simulink model "TRN_test"  (R2022a)
settings: Solver=FixedStepDiscrete  StartTime=0.0  StopTime=300  FixedStep=0.04  RelTol=1e-3
PreLoadFcn:
  | listing = dir;
  | if (contains([listing .name], 'FLCC')) && (contains([listing .name], 'DYN'))
  |     addpath('./DYN', './FLCC', './FTG', './GPS', './INS', './MAP', './RALT', '../TRN');
  | elseif (contains([listing .name], 'FTG.slx'))
  |     addpath('../DYN', '../FLCC', '../FTG', '../GPS', '../INS', '../MAP', '../RALT', '../TRN');
  | else
  | 
  | end
  | 
  | load('BUS_STRUCTURE_DYN.mat');
  | load('BUS_STRUCTURE_FLCC.mat');
  | load('BUS_STRUCTURE_RALT.mat');
  | load('BUS_STRUCTURE_INS.mat');
  | load('BUS_STRUCTURE_GPS.mat');
  | FTG_initState;
  | 
  | addpath('C:/MAP2');
InitFcn:
  | addpath('C:/MAP2');
  | load('BusStructureTRN.mat');
model workspace (MAT data in the model file):
  initLLA = [0 0 0]
libraries: aerolibconvert2 x14, simulink_extras x8
settings Model: ParameterArgumentNames=initLLA  Creator=HSU  LastModifiedBy=JSLee
settings SolverCC: AlgebraicLoopSolver=TrustRegion
settings DataIOCC: ExternalInput=FTGScenario.getElement('IN_STICK'),[],[],FTGScenario.getElement('IN_FLIGHT_CMD'),[]  LoadExternalInput=on  SaveOutput=off  DSMLogging=off  SaveTime=off
settings OptimizationCC: BlockReduction=off  DefaultParameterBehavior=Inlined  UseDivisionForNetSlopeComputation=on  GainParamInheritBuiltInType=on  UseFloatMulNetSlope=on  InlineInvariantSignals=on  EnhancedBackFolding=on  PassReuseOutputArgsAs=Individual arguments  ZeroExternalMemoryAtStartup=off  ZeroInternalMemoryAtStartup=off  NoFixptDivByZeroProtection=on  EfficientFloat2IntCast=on  OptimizeBlockOrder=speed  DifferentSizesBufferReuse=on  OptimizationCustomize=off  EfficientTunableParamExpr=on
settings DebuggingCC: ParameterTunabilityLossMsg=error  UnconnectedInputMsg=warning  UnconnectedOutputMsg=warning  UnconnectedLineMsg=warning  SFUnusedDataAndEventsDiag=none  SFUnexpectedBacktrackingDiag=warning  SFNoUnconditionalDefaultTransitionDiag=warning  SFMachineParentedDataDiag=warning
settings HardwareCC: ProdBitPerPointer=32  ProdBitPerSizeT=32  ProdBitPerPtrDiffT=32  ProdLargestAtomicInteger=Long  ProdLargestAtomicFloat=Double  ProdEndianess=BigEndian  ProdWordSize=32  ProdLongLongMode=on  ProdHWDeviceType=Freescale->MPC83xx
settings ModelReferenceCC: ModelReferenceNumInstancesAllowed=Single
settings SFSimCC: SimCustomHeaderCode="#include \"MAP.h\""  SimUserSources=MAP.c  SimUserLibraries=WS2_32.LIB  MATLABDynamicMemAlloc=off
settings RTWCC: Description=Create Visual C/C++ Solution File for Embedded Coder  SystemTargetFile=ert.tlc  GenCodeOnly=on  TemplateMakefile=RTW.MSVCBuild  GenerateReport=on  RTWUseSimCustomCode=on  CustomHeaderCode="#include \"MAP.h\""  CustomSource=MAP.c  CustomLibrary=WS2_32.LIB  BuildConfiguration=Debug  LaunchReport=on  DLArmComputeVersion=19.05
settings CodeAppCC: ForceParamTrailComments=on  IgnoreCustomStorageClasses=off  OperatorAnnotations=on  SimulinkDataObjDesc=on  SFDataObjDesc=on  InsertBlockDesc=on  EnableCustomComments=on
settings ERTTargetCC: TargetLangStandard=C99 (ISO)  GenerateSampleERTMain=on  InlinedParameterPlacement=NonHierarchical  ERTCustomFileTemplate=example_file_process.tlc

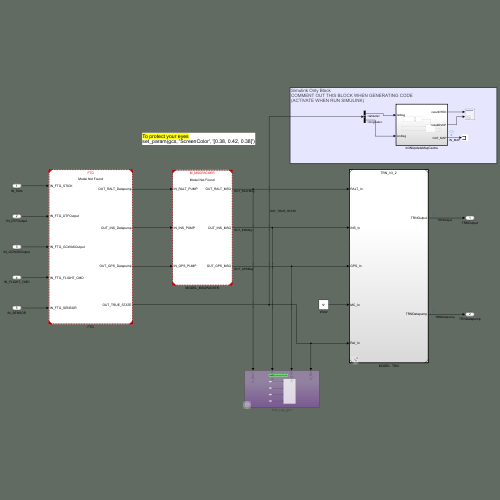
[thumbnail: Simulink's stored preview of the top-level diagram]
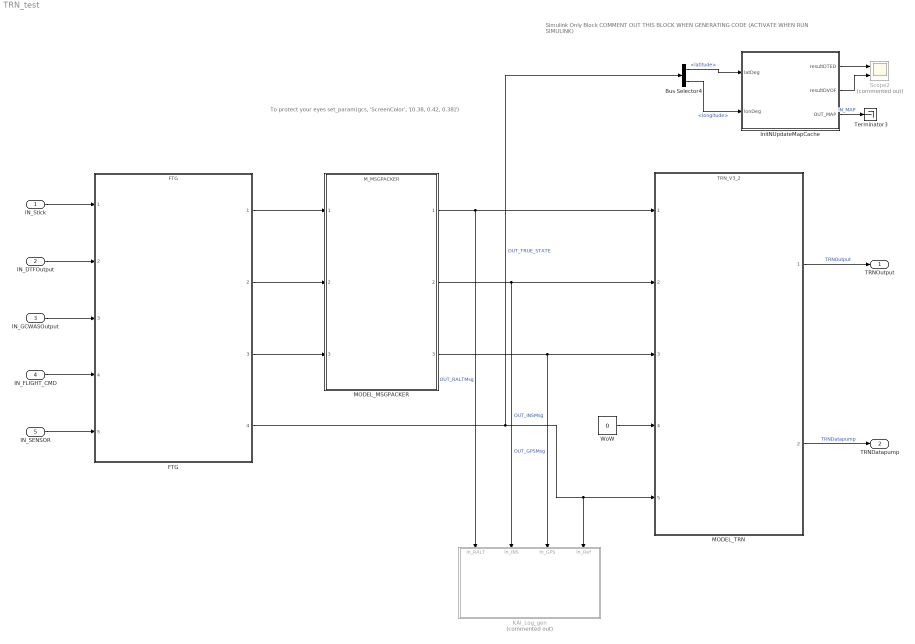
== system TRN_test ==
  note: To protect your eyes
      | set_param(gcs, 'ScreenColor', '[0.38, 0.42, 0.38]')
  note: Simulink Only Block
      | COMMENT OUT THIS BLOCK WHEN GENERATING CODE
      | (ACTIVATE WHEN RUN SIMULINK)
  IN_Stick : Inport  OutDataTypeStr=Bus: BUS_FLCC_STICK
  IN_DTFOutput : Inport  Port=2  OutDataTypeStr=Bus: DTFOutput
  IN_GCWASOutput : Inport  Port=3  OutDataTypeStr=Bus: GCAWSOutput
  IN_FLIGHT_CMD : Inport  Port=4  OutDataTypeStr=Bus: BUS_FLCC_FLIGHT_CMD
  IN_SENSOR : Inport  Port=5  OutDataTypeStr=Bus: BUS_SENSOR_ALL_INPUTSTATUS  Interpolate=off  BusOutputAsStruct=on
  Bus Selector4 : BusSelector  OutputSignals=latitude,longitude
  FTG : ModelReference  ModelNameDialog=FTG.slx  SimulationMode=Normal  ModelReferenceVersion=1.497
  InitNUpdateMapCache : Subsystem  TreatAsAtomicUnit=on
  KAI_Log_gen : Subsystem  Commented=on
  MODEL_MSGPACKER : ModelReference  ModelNameDialog=M_MSGPACKER.slx  SimulationMode=Normal  ModelReferenceVersion=1.294
  MODEL_TRN : ModelReference  ModelNameDialog=TRN_V3_2.slx  SimulationMode=Normal  ModelReferenceVersion=2.550
  Scope2 : Scope  Commented=on  NumInputPorts=2
  Terminator3 : Terminator
  WoW : Constant  Value=0  OutDataTypeStr=Bus: TRN_MC
  TRNOutput : Outport  OutDataTypeStr=Bus: TRNOutput  VectorParamsAs1DForOutWhenUnconnected=off  BusOutputAsStruct=on
  TRNDatapump : Outport  Port=2  OutDataTypeStr=Bus: TRNDatapump  VectorParamsAs1DForOutWhenUnconnected=off  BusOutputAsStruct=on
  wires:
  FTG/1 -> MODEL_MSGPACKER/1
  FTG/3 -> MODEL_MSGPACKER/3
  IN_FLIGHT_CMD/1 -> FTG/4
  IN_Stick/1 -> FTG/1
  IN_GCWASOutput/1 -> FTG/3
  IN_DTFOutput/1 -> FTG/2
  FTG/2 -> MODEL_MSGPACKER/2
  Bus Selector4/1 -> InitNUpdateMapCache/1(latDeg)  "<latitude>"
  FTG/4 -> Bus Selector4/1, MODEL_TRN/5, KAI_Log_gen/4(In_Ref)  "OUT_TRUE_STATE"
  InitNUpdateMapCache/3(OUT_MAP) -> Terminator3/1  "IN_MAP"
  Bus Selector4/2 -> InitNUpdateMapCache/2(lonDeg)  "<longitude>"
  InitNUpdateMapCache/1(resultDTED) -> Scope2/1
  InitNUpdateMapCache/2(resultDVOF) -> Scope2/2
  MODEL_MSGPACKER/1 -> MODEL_TRN/1, KAI_Log_gen/1(In_RALT)  "OUT_RALTMsg"
  MODEL_MSGPACKER/2 -> MODEL_TRN/2, KAI_Log_gen/2(In_INS)  "OUT_INSMsg"
  MODEL_MSGPACKER/3 -> MODEL_TRN/3, KAI_Log_gen/3(In_GPS)  "OUT_GPSMsg"
  IN_SENSOR/1 -> FTG/5
  MODEL_TRN/1 -> TRNOutput/1  "TRNOutput"
  MODEL_TRN/2 -> TRNDatapump/1  "TRNDatapump"
  WoW/1 -> MODEL_TRN/4

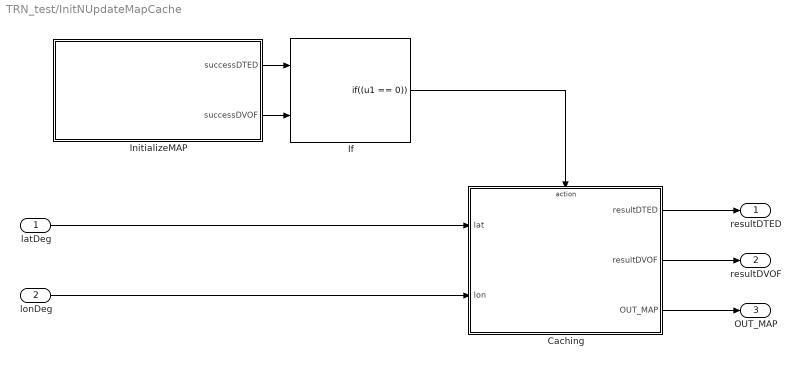
== system TRN_test/InitNUpdateMapCache ==
  latDeg : Inport  OutDataTypeStr=double
  lonDeg : Inport  Port=2  OutDataTypeStr=double
  Caching : Subsystem  TreatAsAtomicUnit=on
  If : If  NumInputs=2  IfExpression=(u1 == 0)  ShowElse=off
  InitializeMAP : MATLAB Function  TreatAsAtomicUnit=on
  resultDTED : Outport  VectorParamsAs1DForOutWhenUnconnected=off
  resultDVOF : Outport  Port=2  VectorParamsAs1DForOutWhenUnconnected=off
  OUT_MAP : Outport  Port=3  OutDataTypeStr=Bus: TRN_MAP
  wires:
  lonDeg/1 -> Caching/2(lon)
  Caching/1(resultDTED) -> resultDTED/1
  InitializeMAP/1(successDTED) -> If/1
  latDeg/1 -> Caching/1(lat)
  Caching/2(resultDVOF) -> resultDVOF/1
  InitializeMAP/2(successDVOF) -> If/2
  If/1 -> Caching/Action
  Caching/3(OUT_MAP) -> OUT_MAP/1

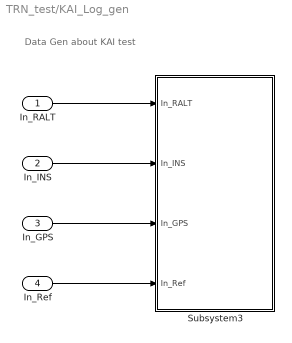
== system TRN_test/KAI_Log_gen ==
  note: Data Gen about KAI test
  In_RALT : Inport
  In_INS : Inport  Port=2
  In_GPS : Inport  Port=3
  In_Ref : Inport  Port=4
  Subsystem3 : Subsystem
  wires:
  In_GPS/1 -> Subsystem3/3(In_GPS)
  In_RALT/1 -> Subsystem3/1(In_RALT)
  In_INS/1 -> Subsystem3/2(In_INS)
  In_Ref/1 -> Subsystem3/4(In_Ref)

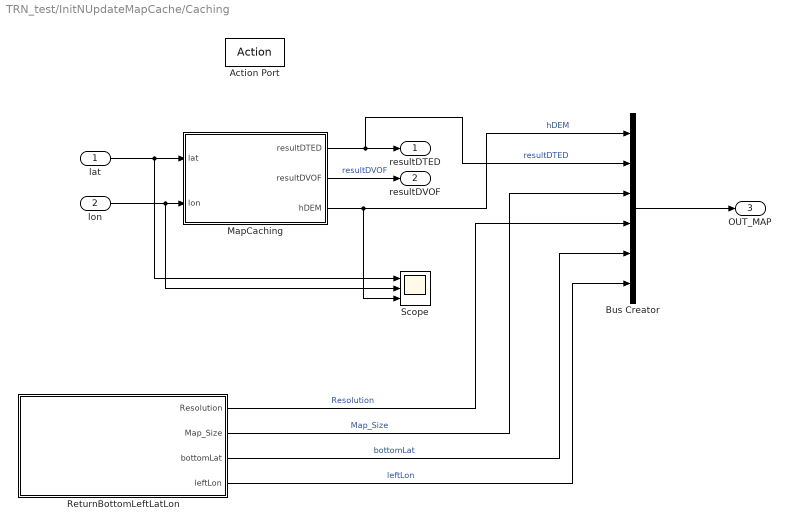
== system TRN_test/InitNUpdateMapCache/Caching ==
  lat : Inport
  lon : Inport  Port=2
  Action Port : ActionPort  ActionPortLabel=if((u1 == 0))
  Bus Creator : BusCreator  Inputs=6  OutDataTypeStr=Bus: TRN_MAP  NonVirtualBus=on
  MapCaching : MATLAB Function  TreatAsAtomicUnit=on
  ReturnBottomLeftLatLon : MATLAB Function  TreatAsAtomicUnit=on
  Scope : Scope  NumInputPorts=3
  resultDTED : Outport  VectorParamsAs1DForOutWhenUnconnected=off
  resultDVOF : Outport  Port=2  VectorParamsAs1DForOutWhenUnconnected=off
  OUT_MAP : Outport  Port=3  OutDataTypeStr=Bus: TRN_MAP
  wires:
  MapCaching/1(resultDTED) -> Bus Creator/2, resultDTED/1  "resultDTED"
  lat/1 -> Scope/1, MapCaching/1(lat)
  lon/1 -> Scope/2, MapCaching/2(lon)
  MapCaching/2(resultDVOF) -> resultDVOF/1  "resultDVOF"
  Bus Creator/1 -> OUT_MAP/1
  ReturnBottomLeftLatLon/2(Map_Size) -> Bus Creator/3  "Map_Size"
  MapCaching/3(hDEM) -> Scope/3, Bus Creator/1  "hDEM"
  ReturnBottomLeftLatLon/1(Resolution) -> Bus Creator/4  "Resolution"
  ReturnBottomLeftLatLon/3(bottomLat) -> Bus Creator/5  "bottomLat"
  ReturnBottomLeftLatLon/4(leftLon) -> Bus Creator/6  "leftLon"

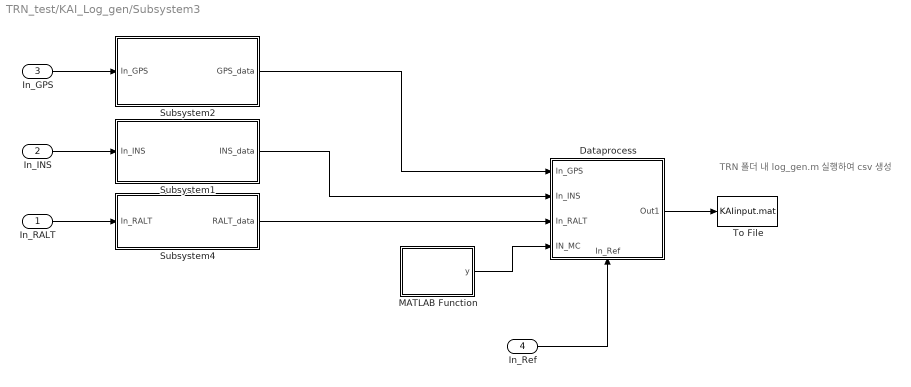
== system TRN_test/KAI_Log_gen/Subsystem3 ==
  note: TRN 폴더 내 log_gen.m 실행하여 csv 생성
  In_RALT : Inport
  In_INS : Inport  Port=2
  In_GPS : Inport  Port=3
  In_Ref : Inport  Port=4
  Dataprocess : Subsystem
      settings: PortSchema="{\"entries\":[{\"content\":{\"sides\":[{\"content\":{\"connectorIds\":[\"In1\",\"In2\",\"In3\",\"In4\"]},\"type\":\"ConnectorPlacement.EquallySpacedRectSide\",\"uuid\":\"447cc120-3690-4207-b031-2a67902aebab\"},{\"content\":{\"connectorIds\":[\"Out1\"],\"side\":\"RIGHT\"},\"type\":\"ConnectorPlacement.EquallySpacedRectSide\",\"uuid\":\"2ef445a1-1f63-4c00-824a-169d2e9bd066\"},{\"content\":{\"connectorIds\":[],\"side\":\"TOP\"},\"type\":\"ConnectorPlacement.EquallySpacedRectSide\",\"uuid\":\"6294caf4-0137-4c2f-b338-5b1e9bc5ecdf\"},{\"content\":{\"connectorIds\":[\"In5\"],\"side\":\"BOTTOM\"},\"type\":\"ConnectorPlacement.EquallySpacedRectSide\",\"uuid\":\"5fdddfb9-1d12-44ef-9d2c-05047e40be8f\"}]},\"type\":\"ConnectorPlacement.EquallySpacedConnector\",\"uuid\":\"5de02e3c-cc0e-487c-ba76-e47ac4ac4be4\"}],\"packageUris\":[\"http://schema.mathworks.com/mf0/Connector/R2020b\"],\"version\":\"1.0\"}"
  MATLAB Function : MATLAB Function  TreatAsAtomicUnit=on
  Subsystem1 : Subsystem
  Subsystem2 : Subsystem
  Subsystem4 : Subsystem
  To File : ToFile  Filename=KAIinput.mat  MatrixName=In_KAIdata  SaveFormat=Timeseries
  wires:
  Subsystem1/1(INS_data) -> Dataprocess/2(In_INS)
  MATLAB Function/1(y) -> Dataprocess/4(IN_MC)
  Subsystem2/1(GPS_data) -> Dataprocess/1(In_GPS)
  In_GPS/1 -> Subsystem2/1(In_GPS)
  In_INS/1 -> Subsystem1/1(In_INS)
  In_RALT/1 -> Subsystem4/1(In_RALT)
  Subsystem4/1(RALT_data) -> Dataprocess/3(In_RALT)
  In_Ref/1 -> Dataprocess/5(In_Ref)
  Dataprocess/1(Out1) -> To File/1

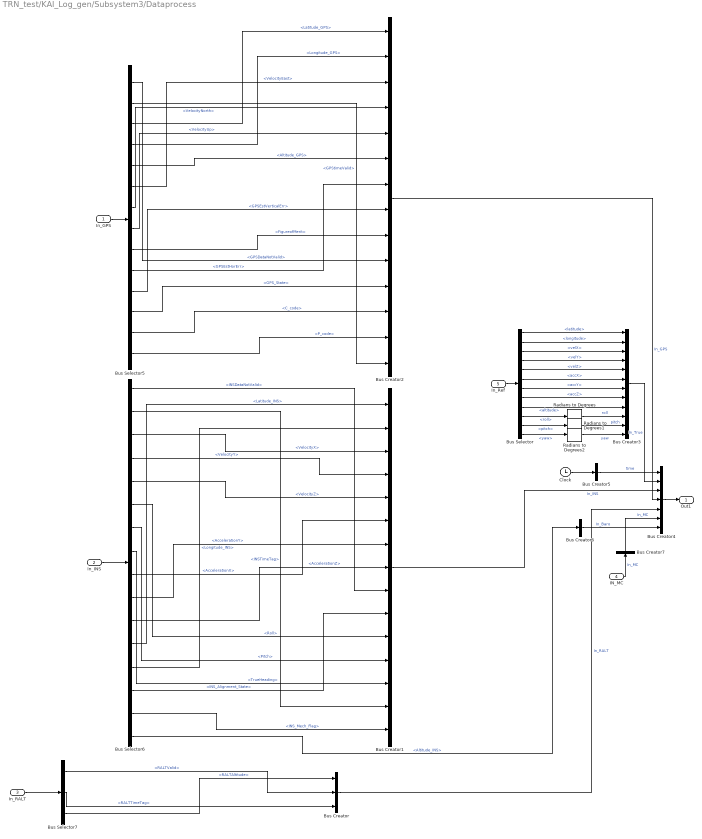
== system TRN_test/KAI_Log_gen/Subsystem3/Dataprocess ==
  In_GPS : Inport
  In_INS : Inport  Port=2
  In_RALT : Inport  Port=3
  IN_MC : Inport  Port=4
  In_Ref : Inport  Port=5
  Bus Creator : BusCreator  Inputs=3
  Bus Creator1 : BusCreator  Inputs=15
  Bus Creator2 : BusCreator  Inputs=14
  Bus Creator3 : BusCreator  Inputs=12
  Bus Creator4 : BusCreator  Inputs=7
  Bus Creator5 : BusCreator  Inputs=1
  Bus Creator6 : BusCreator  Inputs=1
  Bus Creator7 : BusCreator  Inputs=1
  Bus Selector : BusSelector  OutputSignals=latitude,longitude,velX,velY,velZ,accX,accY,accZ,altitude,roll,pitch,yaw
  Bus Selector5 : BusSelector  OutputSignals=GPSDataNotValid,GPStimeValid,Latitude_GPS,Longitude_GPS,Altitude_GPS,VelocityEast,VelocityNorth,VelocityUp,FigureofMerit,GPSEstHorErr,GPSEstVerticalErr,GPS_State,C_code,P_code
  Bus Selector6 : BusSelector  OutputSignals=INSDataNotValid,INSTimeTag,VelocityX,VelocityY,VelocityZ,Roll,Pitch,TrueHeading,AccelerationX,AccelerationY,AccelerationZ,Latitude_INS,Longitude_INS,INS_Alignment_State,INS_Mech_Flag,Altitude_INS
  Bus Selector7 : BusSelector  OutputSignals=RALTValid,RALTTimeTag,RALTAltitude
  Clock : Clock
  Radians to Degrees : simulink_extras/Transformations/Radians to Degrees
  Radians to Degrees1 : simulink_extras/Transformations/Radians to Degrees
  Radians to Degrees2 : simulink_extras/Transformations/Radians to Degrees
  Out1 : Outport
  wires:
  Bus Selector5/8 -> Bus Creator2/5  "<VelocityUp>"
  Bus Selector6/14 -> Bus Creator1/10  "<INS_Alignment_State>"
  Bus Selector5/7 -> Bus Creator2/4  "<VelocityNorth>"
  In_GPS/1 -> Bus Selector5/1
  Bus Selector5/4 -> Bus Creator2/2  "<Longitude_GPS>"
  Bus Selector5/11 -> Bus Creator2/8  "<GPSEstVerticalErr>"
  Bus Selector5/3 -> Bus Creator2/1  "<Latitude_GPS>"
  Bus Selector6/12 -> Bus Creator1/1  "<Latitude_INS>"
  Bus Selector6/13 -> Bus Creator1/2  "<Longitude_INS>"
  Bus Selector5/12 -> Bus Creator2/11  "<GPS_State>"
  Bus Selector6/8 -> Bus Creator1/13  "<TrueHeading>"
  Bus Selector5/14 -> Bus Creator2/13  "<P_code>"
  Bus Selector6/1 -> Bus Creator1/9  "<INSDataNotValid>"
  Bus Selector5/6 -> Bus Creator2/3  "<VelocityEast>"
  Bus Selector6/11 -> Bus Creator1/8  "<AccelerationZ>"
  Bus Selector6/3 -> Bus Creator1/3  "<VelocityX>"
  Bus Selector5/13 -> Bus Creator2/12  "<C_code>"
  Bus Selector5/5 -> Bus Creator2/6  "<Altitude_GPS>"
  Bus Selector6/9 -> Bus Creator1/6  "<AccelerationX>"
  Bus Selector7/3 -> Bus Creator/1  "<RALTAltitude>"
  Bus Selector7/1 -> Bus Creator/2  "<RALTValid>"
  Bus Selector5/1 -> Bus Creator2/10  "<GPSDataNotValid>"
  Bus Selector6/15 -> Bus Creator1/15  "<INS_Mech_Flag>"
  Bus Selector6/4 -> Bus Creator1/4  "<VelocityY>"
  Bus Selector6/6 -> Bus Creator1/11  "<Roll>"
  Bus Selector7/2 -> Bus Creator/3  "<RALTTimeTag>"
  Bus Selector6/5 -> Bus Creator1/5  "<VelocityZ>"
  Bus Selector6/2 -> Bus Creator1/14  "<INSTimeTag>"
  Bus Selector6/7 -> Bus Creator1/12  "<Pitch>"
  Bus Selector5/2 -> Bus Creator2/14  "<GPStimeValid>"
  Bus Selector5/10 -> Bus Creator2/7  "<GPSEstHorErr>"
  Bus Selector6/10 -> Bus Creator1/7  "<AccelerationY>"
  Bus Selector5/9 -> Bus Creator2/9  "<FigureofMerit>"
  In_RALT/1 -> Bus Selector7/1
  In_INS/1 -> Bus Selector6/1
  In_Ref/1 -> Bus Selector/1
  Bus Selector/1 -> Bus Creator3/1  "<latitude>"
  Bus Selector/2 -> Bus Creator3/2  "<longitude>"
  Bus Selector/3 -> Bus Creator3/3  "<velX>"
  Bus Selector/4 -> Bus Creator3/4  "<velY>"
  Bus Selector/5 -> Bus Creator3/5  "<velZ>"
  Bus Selector/6 -> Bus Creator3/6  "<accX>"
  Bus Selector/7 -> Bus Creator3/7  "<accY>"
  Bus Selector/8 -> Bus Creator3/8  "<accZ>"
  Bus Selector/9 -> Bus Creator3/9  "<altitude>"
  Bus Selector/10 -> Radians to Degrees/1  "<roll>"
  Bus Selector/11 -> Radians to Degrees1/1  "<pitch>"
  Bus Selector/12 -> Radians to Degrees2/1  "<yaw>"
  Radians to Degrees/1 -> Bus Creator3/10  "roll"
  Radians to Degrees1/1 -> Bus Creator3/11  "pitch"
  Radians to Degrees2/1 -> Bus Creator3/12  "yaw"
  Bus Creator3/1 -> Bus Creator4/2  "In_True"
  Bus Creator1/1 -> Bus Creator4/3  "In_INS"
  Bus Creator2/1 -> Bus Creator4/4  "In_GPS"
  Bus Creator/1 -> Bus Creator4/5  "In_RALT"
  Bus Creator4/1 -> Out1/1
  Clock/1 -> Bus Creator5/1
  Bus Creator5/1 -> Bus Creator4/1  "time"
  Bus Creator6/1 -> Bus Creator4/7  "In_Baro"
  Bus Creator7/1 -> Bus Creator4/6  "In_MC"
  Bus Selector6/16 -> Bus Creator6/1  "<Altitude_INS>"
  IN_MC/1 -> Bus Creator7/1  "In_MC"

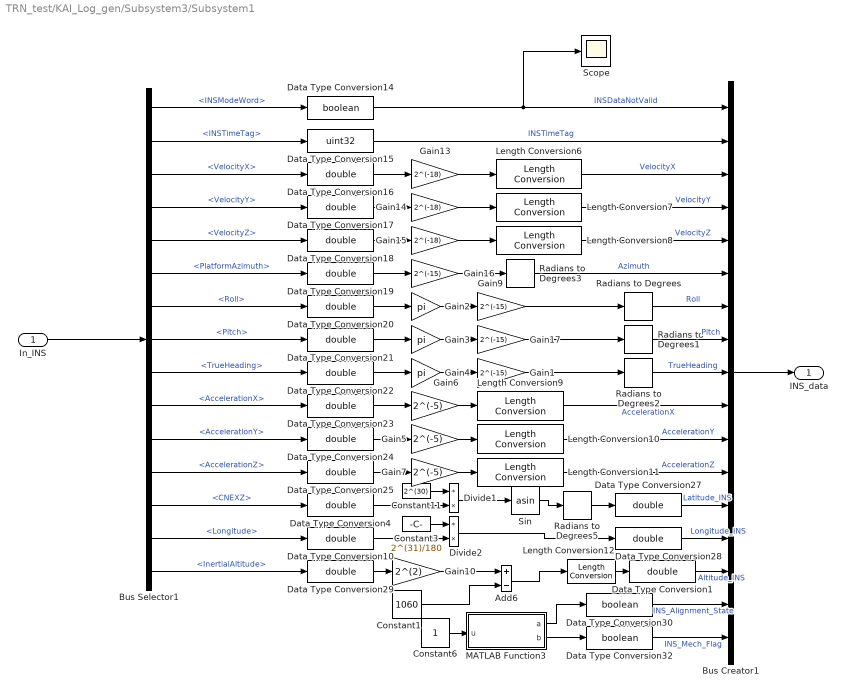
== system TRN_test/KAI_Log_gen/Subsystem3/Subsystem1 ==
  In_INS : Inport
  Add6 : Sum  Inputs=+-
  Bus Creator1 : BusCreator  Inputs=17  OutDataTypeStr=Bus: TRN_INS
  Bus Selector1 : BusSelector  OutputSignals=INSModeWord,INSTimeTag,VelocityX,VelocityY,VelocityZ,PlatformAzimuth,Roll,Pitch,TrueHeading,AccelerationX,AccelerationY,AccelerationZ,CNEXZ,Longitude,InertialAltitude
  Constant1 : Constant  Value=1060
  Constant11 : Constant  Value=2^(30)
  Constant3 : Constant  Value=2^(31)/180
  Constant6 : Constant
  Data Type Conversion{1,4,10,16..25,27..29} (16 alike) : DataTypeConversion  OutDataTypeStr=double  SaturateOnIntegerOverflow=off  RndMeth=Floor
  Data Type Conversion14 : DataTypeConversion  OutDataTypeStr=boolean  SaturateOnIntegerOverflow=off  RndMeth=Floor
  Data Type Conversion15 : DataTypeConversion  OutDataTypeStr=uint32  SaturateOnIntegerOverflow=off  RndMeth=Floor
  Data Type Conversion30 : DataTypeConversion  OutDataTypeStr=boolean  SaturateOnIntegerOverflow=off  RndMeth=Floor
  Data Type Conversion32 : DataTypeConversion  OutDataTypeStr=boolean  SaturateOnIntegerOverflow=off  RndMeth=Floor
  Divide1 : Product  Inputs=/*
  Divide2 : Product  Inputs=/*
  Gain{1,9,16..17} (4 alike) : Gain  Gain=2^(-15)
  Gain10 : Gain  Gain=2^(2)
  Gain13 : Gain  Gain=2^(-18)
  Gain14 : Gain  Gain=2^(-18)
  Gain15 : Gain  Gain=2^(-18)
  Gain2 : Gain  Gain=pi
  Gain3 : Gain  Gain=pi
  Gain4 : Gain  Gain=pi
  Gain5 : Gain  Gain=2^(-5)
  Gain6 : Gain  Gain=2^(-5)
  Gain7 : Gain  Gain=2^(-5)
  Length Conversion{6..12} (7 alike) : aerolibconvert2/Length Conversion  IU=ft  OU=m
  MATLAB Function3 : MATLAB Function  TreatAsAtomicUnit=on
  Radians to Degrees{,1..3,5} (5 alike) : simulink_extras/Transformations/Radians to Degrees
  Scope : Scope
  Sin : Trigonometry  Operator=asin
  INS_data : Outport
  wires:
  Length Conversion6/1 -> Bus Creator1/3  "VelocityX"
  Constant6/1 -> MATLAB Function3/1(u)
  MATLAB Function3/2(b) -> Data Type Conversion32/1
  Data Type Conversion32/1 -> Bus Creator1/17  "INS_Mech_Flag"
  Data Type Conversion22/1 -> Gain4/1
  Length Conversion9/1 -> Bus Creator1/10  "AccelerationX"
  Data Type Conversion29/1 -> Gain10/1
  Radians to Degrees2/1 -> Bus Creator1/9  "TrueHeading"
  Data Type Conversion16/1 -> Gain13/1
  Data Type Conversion28/1 -> Bus Creator1/14  "Longitude_INS"
  Data Type Conversion18/1 -> Gain15/1
  Data Type Conversion15/1 -> Bus Creator1/2  "INSTimeTag"
  Bus Selector1/14 -> Data Type Conversion10/1  "<Longitude>"
  Radians to Degrees5/1 -> Data Type Conversion27/1
  Data Type Conversion24/1 -> Gain5/1
  Sin/1 -> Radians to Degrees5/1
  Constant1/1 -> Add6/2
  Gain14/1 -> Length Conversion7/1
  Data Type Conversion14/1 -> Scope/1, Bus Creator1/1  "INSDataNotValid"
  Bus Selector1/5 -> Data Type Conversion18/1  "<VelocityZ>"
  Data Type Conversion25/1 -> Gain7/1
  Divide2/1 -> Data Type Conversion28/1
  MATLAB Function3/1(a) -> Data Type Conversion30/1
  Data Type Conversion19/1 -> Gain16/1
  Bus Selector1/10 -> Data Type Conversion23/1  "<AccelerationX>"
  Data Type Conversion20/1 -> Gain2/1
  Bus Selector1/6 -> Data Type Conversion19/1  "<PlatformAzimuth>"
  Data Type Conversion27/1 -> Bus Creator1/13  "Latitude_INS"
  Data Type Conversion23/1 -> Gain6/1
  Bus Selector1/7 -> Data Type Conversion20/1  "<Roll>"
  Bus Selector1/2 -> Data Type Conversion15/1  "<INSTimeTag>"
  Bus Selector1/4 -> Data Type Conversion17/1  "<VelocityY>"
  Bus Selector1/3 -> Data Type Conversion16/1  "<VelocityX>"
  Add6/1 -> Length Conversion12/1
  Bus Selector1/15 -> Data Type Conversion29/1  "<InertialAltitude>"
  Bus Selector1/12 -> Data Type Conversion25/1  "<AccelerationZ>"
  Bus Selector1/13 -> Data Type Conversion4/1  "<CNEXZ>"
  Data Type Conversion4/1 -> Divide1/2
  Bus Selector1/9 -> Data Type Conversion22/1  "<TrueHeading>"
  Gain15/1 -> Length Conversion8/1
  Bus Selector1/11 -> Data Type Conversion24/1  "<AccelerationY>"
  Length Conversion12/1 -> Data Type Conversion1/1
  Gain6/1 -> Length Conversion9/1
  Data Type Conversion21/1 -> Gain3/1
  Length Conversion8/1 -> Bus Creator1/5  "VelocityZ"
  Data Type Conversion17/1 -> Gain14/1
  Radians to Degrees1/1 -> Bus Creator1/8  "Pitch"
  Length Conversion7/1 -> Bus Creator1/4  "VelocityY"
  Constant3/1 -> Divide2/1
  Gain5/1 -> Length Conversion10/1
  Length Conversion10/1 -> Bus Creator1/11  "AccelerationY"
  Gain7/1 -> Length Conversion11/1
  Radians to Degrees/1 -> Bus Creator1/7  "Roll"
  Divide1/1 -> Sin/1
  Bus Selector1/8 -> Data Type Conversion21/1  "<Pitch>"
  Data Type Conversion10/1 -> Divide2/2
  Data Type Conversion30/1 -> Bus Creator1/16  "INS_Alignment_State"
  Gain10/1 -> Add6/1
  Radians to Degrees3/1 -> Bus Creator1/6  "Azimuth"
  Length Conversion11/1 -> Bus Creator1/12  "AccelerationZ"
  Constant11/1 -> Divide1/1
  Gain16/1 -> Radians to Degrees3/1
  Gain13/1 -> Length Conversion6/1
  Bus Creator1/1 -> INS_data/1
  In_INS/1 -> Bus Selector1/1
  Gain3/1 -> Gain17/1
  Gain4/1 -> Gain1/1
  Gain2/1 -> Gain9/1
  Gain9/1 -> Radians to Degrees/1
  Gain17/1 -> Radians to Degrees1/1
  Gain1/1 -> Radians to Degrees2/1
  Bus Selector1/1 -> Data Type Conversion14/1  "<INSModeWord>"
  Data Type Conversion1/1 -> Bus Creator1/15  "Altitude_INS"

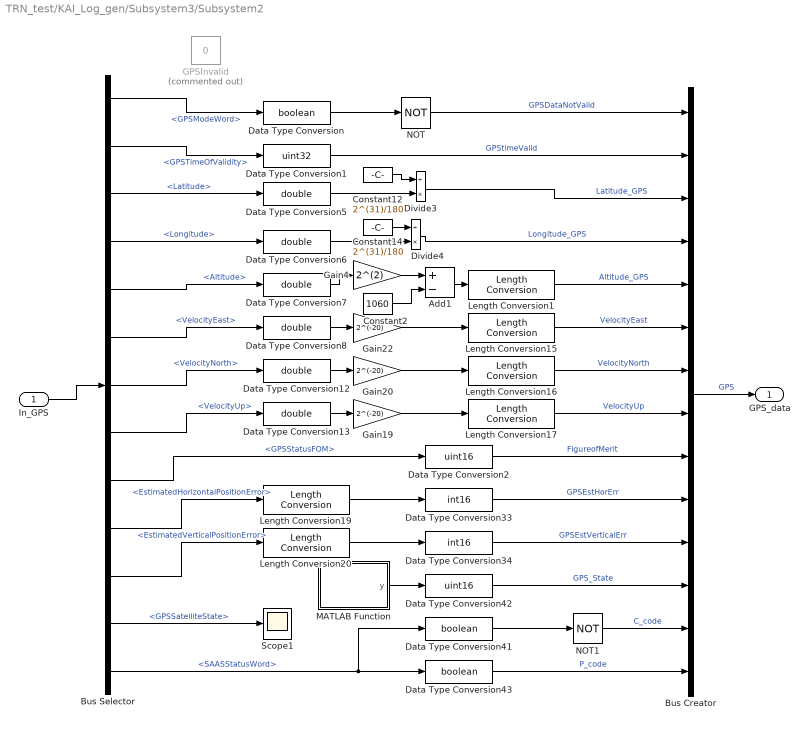
== system TRN_test/KAI_Log_gen/Subsystem3/Subsystem2 ==
  In_GPS : Inport
  Add1 : Sum  Inputs=+-
  Bus Creator : BusCreator  Inputs=14  OutDataTypeStr=Bus: TRN_GPS
  Bus Selector : BusSelector  OutputSignals=GPSModeWord,GPSTimeOfValidity,Latitude,Longitude,Altitude,VelocityEast,VelocityNorth,VelocityUp,GPSStatusFOM,EstimatedHorizontalPositionError,EstimatedVerticalPositionError,GPSSatelliteState,SAASStatusWord
  Constant12 : Constant  Value=2^(31)/180
  Constant14 : Constant  Value=2^(31)/180
  Constant2 : Constant  Value=1060
  Data Type Conversion : DataTypeConversion  OutDataTypeStr=boolean  SaturateOnIntegerOverflow=off  RndMeth=Floor
  Data Type Conversion1 : DataTypeConversion  OutDataTypeStr=uint32  SaturateOnIntegerOverflow=off  RndMeth=Floor
  Data Type Conversion{5..8,12..13} (6 alike) : DataTypeConversion  OutDataTypeStr=double  SaturateOnIntegerOverflow=off  RndMeth=Floor
  Data Type Conversion2 : DataTypeConversion  OutDataTypeStr=uint16  SaturateOnIntegerOverflow=off  RndMeth=Floor
  Data Type Conversion33 : DataTypeConversion  OutDataTypeStr=int16  SaturateOnIntegerOverflow=off  RndMeth=Floor
  Data Type Conversion34 : DataTypeConversion  OutDataTypeStr=int16  SaturateOnIntegerOverflow=off  RndMeth=Floor
  Data Type Conversion41 : DataTypeConversion  OutDataTypeStr=boolean  SaturateOnIntegerOverflow=off  RndMeth=Floor
  Data Type Conversion42 : DataTypeConversion  OutDataTypeStr=uint16  SaturateOnIntegerOverflow=off  RndMeth=Floor
  Data Type Conversion43 : DataTypeConversion  OutDataTypeStr=boolean  SaturateOnIntegerOverflow=off  RndMeth=Floor
  Divide3 : Product  Inputs=/*
  Divide4 : Product  Inputs=/*
  GPSInvalid : Constant  Commented=on  Value=0
  Gain19 : Gain  Gain=2^(-20)
  Gain20 : Gain  Gain=2^(-20)
  Gain22 : Gain  Gain=2^(-20)
  Gain4 : Gain  Gain=2^(2)
  Length Conversion{1,15..17,19..20} (6 alike) : aerolibconvert2/Length Conversion  IU=ft  OU=m
  MATLAB Function : MATLAB Function  TreatAsAtomicUnit=on
  NOT : Logic  Operator=NOT  IconShape=distinctive  AllPortsSameDT=off  OutDataTypeStr=boolean
  NOT1 : Logic  Operator=NOT  IconShape=distinctive  AllPortsSameDT=off  OutDataTypeStr=boolean
  Scope1 : Scope
  GPS_data : Outport
  wires:
  Length Conversion1/1 -> Bus Creator/5  "Altitude_GPS"
  Bus Selector/7 -> Data Type Conversion12/1  "<VelocityNorth>"
  Bus Selector/2 -> Data Type Conversion1/1  "<GPSTimeOfValidity>"
  Bus Selector/3 -> Data Type Conversion5/1  "<Latitude>"
  Gain4/1 -> Add1/1
  Data Type Conversion33/1 -> Bus Creator/10  "GPSEstHorErr"
  Bus Selector/5 -> Data Type Conversion7/1  "<Altitude>"
  Data Type Conversion8/1 -> Gain22/1
  Data Type Conversion41/1 -> NOT1/1
  Bus Selector/11 -> Length Conversion20/1  "<EstimatedVerticalPositionError>"
  Gain20/1 -> Length Conversion16/1
  Bus Selector/10 -> Length Conversion19/1  "<EstimatedHorizontalPositionError>"
  Divide3/1 -> Bus Creator/3  "Latitude_GPS"
  Bus Selector/6 -> Data Type Conversion8/1  "<VelocityEast>"
  Data Type Conversion13/1 -> Gain19/1
  Data Type Conversion6/1 -> Divide4/2
  Data Type Conversion34/1 -> Bus Creator/11  "GPSEstVerticalErr"
  Data Type Conversion42/1 -> Bus Creator/12  "GPS_State"
  Gain22/1 -> Length Conversion15/1
  Length Conversion20/1 -> Data Type Conversion34/1
  Data Type Conversion5/1 -> Divide3/2
  Add1/1 -> Length Conversion1/1
  Data Type Conversion1/1 -> Bus Creator/2  "GPStimeValid"
  Gain19/1 -> Length Conversion17/1
  Data Type Conversion/1 -> NOT/1
  Data Type Conversion2/1 -> Bus Creator/9  "FigureofMerit"
  Data Type Conversion7/1 -> Gain4/1
  Bus Selector/8 -> Data Type Conversion13/1  "<VelocityUp>"
  Bus Selector/4 -> Data Type Conversion6/1  "<Longitude>"
  Bus Selector/9 -> Data Type Conversion2/1  "<GPSStatusFOM>"
  Length Conversion17/1 -> Bus Creator/8  "VelocityUp"
  Length Conversion16/1 -> Bus Creator/7  "VelocityNorth"
  Bus Creator/1 -> GPS_data/1  "GPS"
  Data Type Conversion12/1 -> Gain20/1
  Constant2/1 -> Add1/2
  Length Conversion15/1 -> Bus Creator/6  "VelocityEast"
  Length Conversion19/1 -> Data Type Conversion33/1
  Divide4/1 -> Bus Creator/4  "Longitude_GPS"
  Bus Selector/13 -> Data Type Conversion41/1, Data Type Conversion43/1  "<SAASStatusWord>"
  In_GPS/1 -> Bus Selector/1
  Constant14/1 -> Divide4/1
  Constant12/1 -> Divide3/1
  Data Type Conversion43/1 -> Bus Creator/14  "P_code"
  NOT/1 -> Bus Creator/1  "GPSDataNotValid"
  Bus Selector/12 -> Scope1/1  "<GPSSatelliteState>"
  Bus Selector/1 -> Data Type Conversion/1  "<GPSModeWord>"
  NOT1/1 -> Bus Creator/13  "C_code"
  MATLAB Function/1(y) -> Data Type Conversion42/1

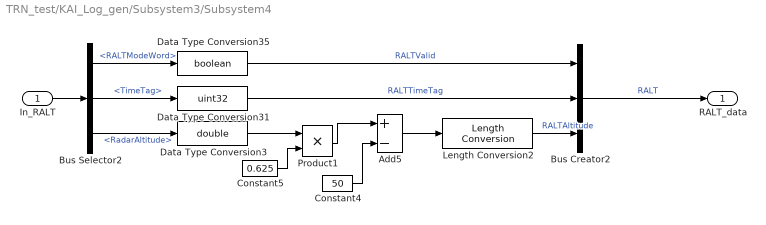
== system TRN_test/KAI_Log_gen/Subsystem3/Subsystem4 ==
  In_RALT : Inport
  Add5 : Sum  Inputs=+-
  Bus Creator2 : BusCreator  Inputs=3  OutDataTypeStr=Bus: TRN_RALT
  Bus Selector2 : BusSelector  OutputSignals=RALTModeWord,TimeTag,RadarAltitude
  Constant4 : Constant  Value=50
  Constant5 : Constant  Value=0.625
  Data Type Conversion3 : DataTypeConversion  OutDataTypeStr=double  SaturateOnIntegerOverflow=off  RndMeth=Floor
  Data Type Conversion31 : DataTypeConversion  OutDataTypeStr=uint32  SaturateOnIntegerOverflow=off  RndMeth=Floor
  Data Type Conversion35 : DataTypeConversion  OutDataTypeStr=boolean  SaturateOnIntegerOverflow=off  RndMeth=Floor
  Length Conversion2 : aerolibconvert2/Length Conversion  IU=ft  OU=m
  Product1 : Product
  RALT_data : Outport
  wires:
  Length Conversion2/1 -> Bus Creator2/3  "RALTAltitude"
  Constant4/1 -> Add5/2
  Bus Creator2/1 -> RALT_data/1  "RALT"
  In_RALT/1 -> Bus Selector2/1
  Data Type Conversion35/1 -> Bus Creator2/1  "RALTValid"
  Add5/1 -> Length Conversion2/1
  Bus Selector2/3 -> Data Type Conversion3/1  "<RadarAltitude>"
  Data Type Conversion3/1 -> Product1/1
  Product1/1 -> Add5/1
  Constant5/1 -> Product1/2
  Data Type Conversion31/1 -> Bus Creator2/2  "RALTTimeTag"
  Bus Selector2/2 -> Data Type Conversion31/1  "<TimeTag>"
  Bus Selector2/1 -> Data Type Conversion35/1  "<RALTModeWord>"

== matlab function TRN_test/InitNUpdateMapCache/Caching/ReturnBottomLeftLatLon ==
  data: Resolution output; Map_Size output; bottomLat output; leftLon output
function [Resolution, Map_Size, bottomLat, leftLon] = ReturnBottomLeftLatLon

Resolution = double(0.0);
Map_Size = double(0.0);

leftLon = 0.0;
% leftLon = coder.ceval('ReturnLeftLon');

bottomLat = 0.0;
% bottomLat = coder.ceval('ReturnBottomLat');

end

== matlab function TRN_test/KAI_Log_gen/Subsystem3/Subsystem2/MATLAB Function ==
  data: y output
function y = fcn

y = 5;

== matlab function TRN_test/KAI_Log_gen/Subsystem3/MATLAB Function ==
  data: y output
function y = fcn

y = boolean(false);

== matlab function TRN_test/KAI_Log_gen/Subsystem3/Subsystem1/MATLAB Function3 ==
  data: u input; a output; b output
function [a,b]  = fcn(u)

% WeightOnWheels
if(u==1)
    a = boolean(true);
    b = boolean(true);
else
    a = boolean(false);
    b = boolean(false);
end

end

== matlab function TRN_test/InitNUpdateMapCache/Caching/MapCaching ==
  data: resultDTED output; resultDVOF output; lat input; lon input; hDEM output
function [resultDTED, resultDVOF, hDEM] = MapCaching(lat, lon)

resultDTED = uint32(1);
resultDVOF = int32(1);
hDEM = double(0.0);                                 %%20220419

% resultDVOF = coder.ceval('UpdateObstList', lat, lon);
% resultDTED = coder.ceval('UpdateMapCache', lat, lon);
hDEM = coder.ceval('MAPGetTerrainHeight', lat, lon);       %%20220419

== matlab function TRN_test/InitNUpdateMapCache/InitializeMAP ==
  data: successDTED output; successDVOF output
function [successDTED, successDVOF] = InitializeMAP()

flagDTED = int32(1);
flagDVOF = int32(1);

pathDTED = 'C:\MAP2\MAP_DB\';
pathDVOF = 'C:\MAP2\DVOF\';

strLenDTED = int32(strlength(pathDTED));
strLenDVOF = int32(strlength(pathDVOF));

flagDTED = coder.ceval('InitialMap', pathDTED, strLenDTED );
% flagDVOF = coder.ceval('InitDVOF', pathDVOF, strLenDVOF );

successDTED = flagDTED;
successDVOF = flagDVOF;
